simulink model "tarea"  (R2023b)
settings: Solver=VariableStepAuto  StartTime=0.0  StopTime=10.0  RelTol=1e-3
settings Model: Creator=Geo  LastModifiedBy=Geo

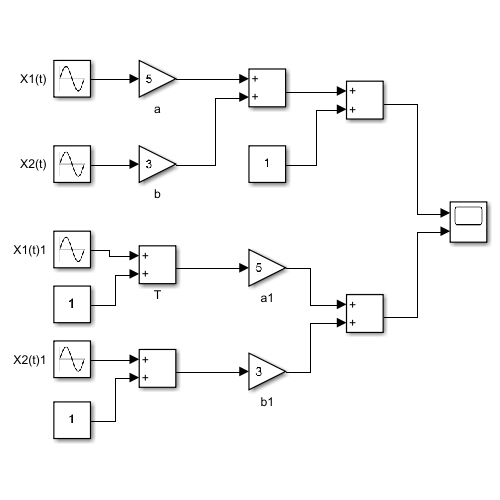
[thumbnail: Simulink's stored preview of the top-level diagram]
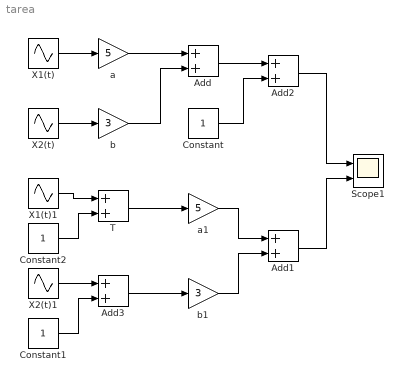
== system tarea ==
  Add{,1..3} (4 alike) : Sum
  Constant : Constant
  Constant1 : Constant
  Constant2 : Constant
  Scope1 : Scope  NumInputPorts=2
  T : Sum
  X1(t) : Sin  SampleTime=0
  X1(t)1 : Sin  SampleTime=0
  X2(t) : Sin  Amplitude=2  SampleTime=0
  X2(t)1 : Sin  Amplitude=2  SampleTime=0
  a : Gain  Gain=5
  a1 : Gain  Gain=5
  b : Gain  Gain=3
  b1 : Gain  Gain=3
  wires:
  X1(t)/1 -> a/1
  X2(t)/1 -> b/1
  a/1 -> Add/1
  b/1 -> Add/2
  Constant/1 -> Add2/2
  Add/1 -> Add2/1
  X2(t)1/1 -> Add3/1
  Constant1/1 -> Add3/2
  X1(t)1/1 -> T/1
  Constant2/1 -> T/2
  Add3/1 -> b1/1
  T/1 -> a1/1
  Add1/1 -> Scope1/2
  a1/1 -> Add1/1
  b1/1 -> Add1/2
  Add2/1 -> Scope1/1
